simulink model "controller"  (R2024b)
settings: Solver=ode45  StartTime=0.0  StopTime=300  RelTol=1e-2
values from neighbouring files (symbols this model uses):
  ss_plant = ss_plant.getMesh()    [HVAC.m]
libraries: cstblocks x1
settings Model: Creator=mikom  LastModifiedBy=mikom

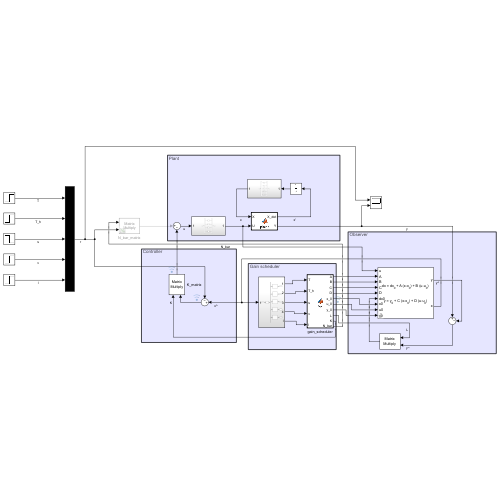
[thumbnail: Simulink's stored preview of the top-level diagram]
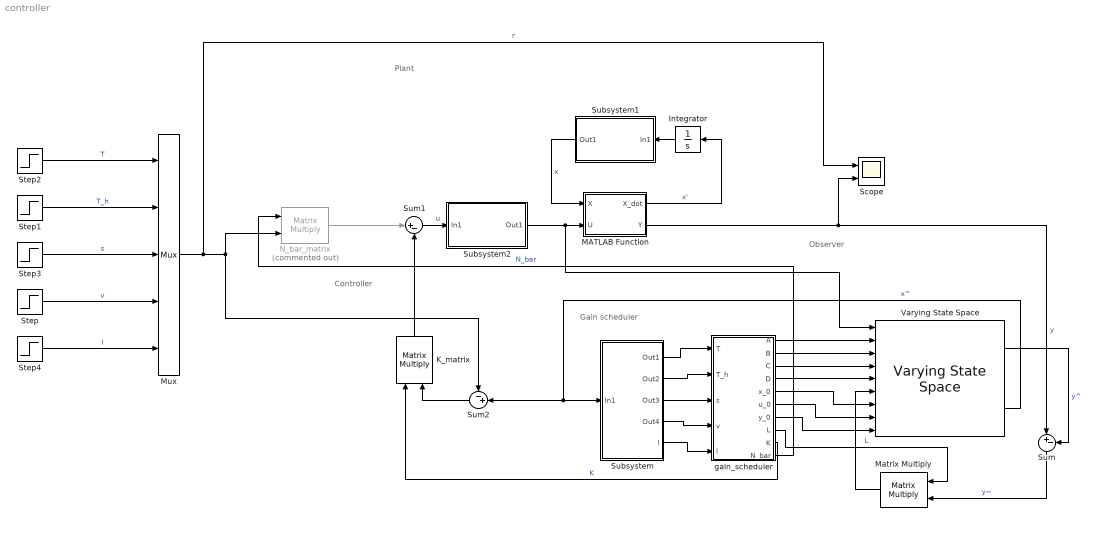
== system controller ==
  note: Controller
  note: Observer
  note: Gain scheduler
  note: Plant
  Integrator : Integrator  InitialCondition=ss_plant.X_init
  K_matrix : Product  Multiplication=Matrix(*)
  MATLAB Function : MATLAB Function  TreatAsAtomicUnit=on
  Matrix Multiply : Product  Multiplication=Matrix(*)
  Mux : Mux  Inputs=5
  N_bar_matrix : Product  Commented=on  Multiplication=Matrix(*)
  Scope : Scope  NumInputPorts=2
  Step : Step  Time=0  Before=0.3  After=0.3  SampleTime=0
  Step1 : Step  Time=0  Before=21  After=21  SampleTime=0
  Step2 : Step  Time=200  Before=25  After=30  SampleTime=0
  Step3 : Step  Time=100  Before=1.5  SampleTime=0
  Step4 : Step  Time=30  Before=2.5  After=5  SampleTime=0
  Subsystem : Subsystem
  Subsystem1 : Subsystem
  Subsystem2 : Subsystem
  Sum : Sum  Inputs=|+-
  Sum1 : Sum  Inputs=|+-
  Sum2 : Sum  Inputs=-+|
  Varying State Space : cstblocks/Linear Parameter Varying/Varying State Space  InitialConditionSource=internal  InitialCondition=ss_plant.X_init  xNames=''  OutputX=on  OutputDX=off  Feedthrough=on  InputX0=on  InputDX0=on  InputU0=on  InputY0=on
  gain_scheduler : MATLAB Function  TreatAsAtomicUnit=on
  wires:
  Step2/1 -> Mux/1  "T"
  Step/1 -> Mux/4  "v"
  Step3/1 -> Mux/3  "s"
  Step1/1 -> Mux/2  "T_h"
  MATLAB Function/2(Y) -> Scope/2, Sum/1  "y"
  MATLAB Function/1(X_dot) -> Integrator/1  "x'"
  Varying State Space/1 -> Sum/2  "y^"
  Integrator/1 -> Subsystem1/1(In1)
  gain_scheduler/1(A) -> Varying State Space/2
  gain_scheduler/2(B) -> Varying State Space/3
  gain_scheduler/3(C) -> Varying State Space/4
  gain_scheduler/4(D) -> Varying State Space/5
  Subsystem/1(Out1) -> gain_scheduler/1(T)
  Subsystem/2(Out2) -> gain_scheduler/2(T_h)
  Subsystem/3(Out3) -> gain_scheduler/3(s)
  Subsystem/4(Out4) -> gain_scheduler/4(v)
  Sum/1 -> Matrix Multiply/2  "y~"
  Varying State Space/2 -> Subsystem/1(In1), Sum2/2  "x^"
  gain_scheduler/6(u_0) -> Varying State Space/8
  gain_scheduler/5(x_0) -> Varying State Space/7
  gain_scheduler/7(y_0) -> Varying State Space/9
  gain_scheduler/8(L) -> Matrix Multiply/1  "L"
  Matrix Multiply/1 -> Varying State Space/6
  gain_scheduler/9(K) -> K_matrix/1  "K"
  K_matrix/1 -> Sum1/2
  Sum1/1 -> Subsystem2/1(In1)  "u"
  Subsystem1/1(Out1) -> MATLAB Function/1(X)  "x"
  Subsystem2/1(Out1) -> Varying State Space/1, MATLAB Function/2(U)
  Step4/1 -> Mux/5  "l"
  Subsystem/5(l) -> gain_scheduler/5(l)
  Sum2/1 -> K_matrix/2
  Mux/1 -> Scope/1, N_bar_matrix/2, Sum2/1  "r"
  gain_scheduler/10(N_bar) -> N_bar_matrix/1  "N_bar"
  N_bar_matrix/1 -> Sum1/1

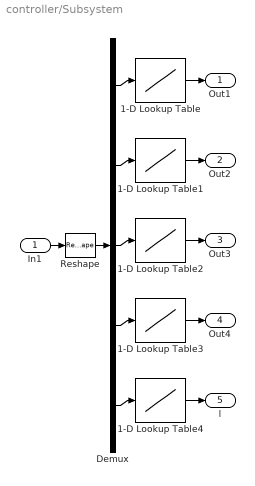
== system controller/Subsystem ==
  In1 : Inport
  1-D Lookup Table : Lookup_n-D  NumberOfTableDimensions=1  BreakpointsForDimension1=ss_plant.breakpoints{1}  Table=[1:1:(size(ss_plant.breakpoints{1},2))]  InterpMethod=Nearest  ExtrapMethod=Clip  InternalRulePriority=Speed  RndMeth=Simplest
  1-D Lookup Table1 : Lookup_n-D  NumberOfTableDimensions=1  BreakpointsForDimension1=ss_plant.breakpoints{2}  Table=[1:1:(size(ss_plant.breakpoints{2},2))]  InterpMethod=Flat  InternalRulePriority=Speed  RndMeth=Simplest
  1-D Lookup Table2 : Lookup_n-D  NumberOfTableDimensions=1  BreakpointsForDimension1=ss_plant.breakpoints{3}  Table=[1:1:(size(ss_plant.breakpoints{3},2))]  InterpMethod=Flat  DiagnosticForOutOfRangeInput=Warning  InternalRulePriority=Speed  RndMeth=Simplest
  1-D Lookup Table3 : Lookup_n-D  NumberOfTableDimensions=1  BreakpointsForDimension1=ss_plant.breakpoints{4}  Table=[1:1:(size(ss_plant.breakpoints{4},2))]  InterpMethod=Nearest  ExtrapMethod=Clip  DiagnosticForOutOfRangeInput=Warning  UseLastTableValue=on  InternalRulePriority=Speed  RndMeth=Simplest
  1-D Lookup Table4 : Lookup_n-D  NumberOfTableDimensions=1  BreakpointsForDimension1=ss_plant.breakpoints{5}  Table=[1:1:(size(ss_plant.breakpoints{5},2))]  InterpMethod=Nearest  ExtrapMethod=Clip  DiagnosticForOutOfRangeInput=Warning  UseLastTableValue=on  InternalRulePriority=Speed  RndMeth=Simplest
  Demux : Demux  Outputs=5
  Reshape : Reshape
  Out1 : Outport
  Out2 : Outport  Port=2
  Out3 : Outport  Port=3
  Out4 : Outport  Port=4
  l : Outport  Port=5
  wires:
  Demux/4 -> 1-D Lookup Table3/1
  Demux/1 -> 1-D Lookup Table/1
  1-D Lookup Table3/1 -> Out4/1
  Demux/3 -> 1-D Lookup Table2/1
  In1/1 -> Reshape/1
  Demux/2 -> 1-D Lookup Table1/1
  1-D Lookup Table1/1 -> Out2/1
  1-D Lookup Table/1 -> Out1/1
  1-D Lookup Table2/1 -> Out3/1
  Reshape/1 -> Demux/1
  Demux/5 -> 1-D Lookup Table4/1
  1-D Lookup Table4/1 -> l/1

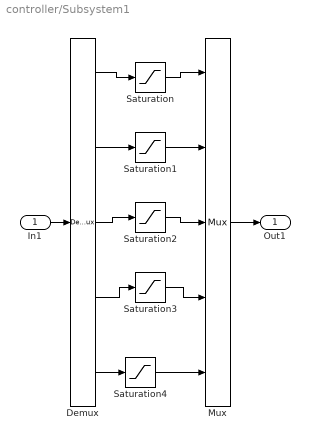
== system controller/Subsystem1 ==
  In1 : Inport
  Demux : Demux  Outputs=5
  Mux : Mux  Inputs=5
  Saturation : Saturate  UpperLimit=1000  LowerLimit=-273.15
  Saturation1 : Saturate  UpperLimit=1000  LowerLimit=-273.15
  Saturation2 : Saturate  UpperLimit=10  LowerLimit=0.2
  Saturation3 : Saturate  UpperLimit=1  LowerLimit=0
  Saturation4 : Saturate  UpperLimit=20  LowerLimit=1.3
  Out1 : Outport
  wires:
  In1/1 -> Demux/1
  Mux/1 -> Out1/1
  Demux/1 -> Saturation/1
  Saturation/1 -> Mux/1
  Demux/2 -> Saturation1/1
  Saturation1/1 -> Mux/2
  Demux/3 -> Saturation2/1
  Saturation2/1 -> Mux/3
  Demux/4 -> Saturation3/1
  Saturation3/1 -> Mux/4
  Demux/5 -> Saturation4/1
  Saturation4/1 -> Mux/5

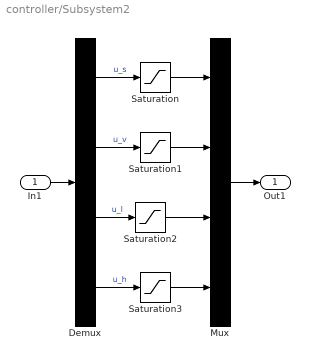
== system controller/Subsystem2 ==
  In1 : Inport
  Demux : Demux
  Mux : Mux
  Saturation : Saturate  UpperLimit=6  LowerLimit=0.2  ZeroCross=off
  Saturation1 : Saturate  UpperLimit=1  LowerLimit=0  ZeroCross=off
  Saturation2 : Saturate  UpperLimit=1  LowerLimit=0  ZeroCross=off
  Saturation3 : Saturate  UpperLimit=1  LowerLimit=0  ZeroCross=off
  Out1 : Outport
  wires:
  In1/1 -> Demux/1
  Mux/1 -> Out1/1
  Demux/1 -> Saturation/1  "u_s"
  Saturation/1 -> Mux/1
  Demux/2 -> Saturation1/1  "u_v"
  Saturation1/1 -> Mux/2
  Saturation2/1 -> Mux/3
  Demux/4 -> Saturation3/1  "u_h"
  Saturation3/1 -> Mux/4
  Demux/3 -> Saturation2/1  "u_l"

== matlab function controller/gain_scheduler ==
  data: T input; A output; T_h input; s input; v input; B output; C output; D output; x_0 output; u_0 output; y_0 output; L output; K output; N_bar output; l input
function [A, B, C, D, x_0, u_0, y_0, L, K, N_bar] = fcn(T,T_h,s,v,l)
    persistent meshData4;
    if isempty(meshData4)
        data = load('mesh.mat', 'mymesh');  % Load only the mesh variable
        meshData4 = data.mymesh;
    end
    mycell = meshData4{T,T_h,s,v,l};
    
    A = mycell.A;
    B = mycell.B;
    C = mycell.C;
    D = mycell.D;
    K = mycell.K;
    L = mycell.L;
    x_0 = mycell.x_0;
    u_0 = mycell.u_0;
    y_0 = mycell.y_0;
    N_bar = mycell.N_bar;
end

== matlab function controller/MATLAB Function ==
  data: X input; X_dot output; U input; Y output
function [X_dot, Y]= plant(X, U)
    [X_dot, Y] = plantFunction(X, U);
end
